simulink model "sampleModel20"  (R2021a)
settings: Solver=VariableStepAuto  StartTime=0.0  StopTime=10.0  RelTol=1e-3
undefined symbols (not defined in the file): DiscIntNeverNeededParam, magnitude, Newton, Raphson
libraries: simulink x274, pid_lib x17
(part 16 of 16)

== system sampleModel20/cfblk97/cfblk3/cfblk10/cfblk7 ==
  cfblk1 : Inport
  cfblk5 : Inport  Port=2
  cfblk6 : Inport  Port=3
  cfblk7 : Inport  Port=4
  cfblk8 : Inport  Port=5
  cfblk9 : Inport  Port=6
  cfblk10 : Inport  Port=7
  cfblk3 : Polyval  Coefs=[ +2.081618890e-019, -1.441693666e-014, +4.719686976e-010, -8.536869453e-006, +1.621573104e-001, -8.087801117e+001 ]
  cfblk4 : Signum
  cfblk2 : Outport
  cfblk11 : Outport  Port=2
  wires:
  cfblk8/1 -> cfblk3/1
  cfblk3/1 -> cfblk2/1
  cfblk4/1 -> cfblk11/1
  cfblk9/1 -> cfblk4/1

== system sampleModel20/cfblk97/cfblk3/cfblk5/cfblk10 ==
  cfblk1 : Inport
  cfblk8 : Inport  Port=2
  cfblk9 : Inport  Port=3
  cfblk10 : Inport  Port=4
  cfblk11 : Inport  Port=5
  cfblk12 : Inport  Port=6
  cfblk13 : Inport  Port=7
  cfblk3 : simulink/Discrete/Transfer Fcn Real Zero  ZeroZ=0.75  ICPrevInput=0.0  DoSatur=off
      settings: SourceProductBaseCode=SL
  cfblk4 : Gain  Gain=[233703993.927434]
  cfblk5 : Reshape
  cfblk6 : Signum
  cfblk7 : Bias  Bias=[437592239.040751]
  cfblk2 : Outport
  cfblk14 : Outport  Port=2
  cfblk15 : Outport  Port=3
  wires:
  cfblk7/1 -> cfblk5/1
  cfblk3/1 -> cfblk7/1
  cfblk1/1 -> cfblk15/1
  cfblk11/1 -> cfblk6/1
  cfblk8/1 -> cfblk4/1
  cfblk12/1 -> cfblk2/1
  cfblk4/1 -> cfblk14/1
  cfblk6/1 -> cfblk3/1

== system sampleModel20/cfblk97/cfblk3/cfblk5/cfblk11 ==
  cfblk1 : Inport
  cfblk6 : Inport  Port=2
  cfblk7 : Inport  Port=3
  cfblk8 : Inport  Port=4
  cfblk3 : simulink/Math Operations/Slider Gain  gain=1  low=0  high=2
  cfblk4 : Gain  Gain=[977320250.884013]
  cfblk5 : Gain  Gain=[-143070157.092891]
  cfblk2 : Outport
  cfblk9 : Outport  Port=2
  wires:
  cfblk8/1 -> cfblk9/1
  cfblk6/1 -> cfblk5/1
  cfblk5/1 -> cfblk4/1
  cfblk7/1 -> cfblk2/1
  cfblk1/1 -> cfblk3/1

== system sampleModel20/cfblk97/cfblk3/cfblk5/cfblk12 ==
  cfblk1 : Inport
  cfblk8 : Inport  Port=2
  cfblk9 : Inport  Port=3
  cfblk10 : Inport  Port=4
  cfblk11 : Inport  Port=5
  cfblk12 : Inport  Port=6
  cfblk13 : Inport  Port=7
  cfblk14 : Inport  Port=8
  cfblk3 : Polyval  Coefs=[ +2.081618890e-019, -1.441693666e-014, +4.719686976e-010, -8.536869453e-006, +1.621573104e-001, -8.087801117e+001 ]
  cfblk4 : Signum
  cfblk5 : Sqrt  Operator=rSqrt  AlgorithmType=Newton-Raphson  SaturateOnIntegerOverflow=on
  cfblk6 : PermuteDimensions
  cfblk7 : Reshape
  cfblk2 : Outport
  cfblk15 : Outport  Port=2
  cfblk16 : Outport  Port=3
  cfblk17 : Outport  Port=4
  wires:
  cfblk13/1 -> cfblk6/1
  cfblk10/1 -> cfblk7/1
  cfblk11/1 -> cfblk16/1
  cfblk6/1 -> cfblk15/1
  cfblk3/1 -> cfblk17/1
  cfblk8/1 -> cfblk3/1
  cfblk5/1 -> cfblk4/1
  cfblk1/1 -> cfblk2/1
  cfblk9/1 -> cfblk5/1

== system sampleModel20/cfblk97/cfblk3/cfblk5/cfblk7 ==
  cfblk1 : Inport
  cfblk6 : Inport  Port=2
  cfblk7 : Inport  Port=3
  cfblk8 : Inport  Port=4
  cfblk9 : Inport  Port=5
  cfblk10 : Inport  Port=6
  cfblk11 : Inport  Port=7
  cfblk12 : Inport  Port=8
  cfblk13 : Inport  Port=9
  cfblk14 : Inport  Port=10
  cfblk3 : Sqrt  SaturateOnIntegerOverflow=on
  cfblk4 : Sqrt  SaturateOnIntegerOverflow=on
  cfblk5 : Gain  Gain=[-337074961.948638]
  cfblk2 : Outport
  wires:
  cfblk4/1 -> cfblk5/1
  cfblk11/1 -> cfblk4/1
  cfblk14/1 -> cfblk3/1
  cfblk1/1 -> cfblk2/1

== system sampleModel20/cfblk97/cfblk3/cfblk5/cfblk8 ==
  cfblk1 : Inport
  cfblk8 : Inport  Port=2
  cfblk9 : Inport  Port=3
  cfblk10 : Inport  Port=4
  cfblk11 : Inport  Port=5
  cfblk12 : Inport  Port=6
  cfblk3 : Product
  cfblk4 : Squeeze
  cfblk5 : Trigonometry
  cfblk6 : Rounding
  cfblk7 : Product
  cfblk2 : Outport
  cfblk13 : Outport  Port=2
  cfblk14 : Outport  Port=3
  cfblk15 : Outport  Port=4
  wires:
  cfblk1/1 -> cfblk4/1
  cfblk7/1 -> cfblk14/1
  cfblk8/1 -> cfblk7/1
  cfblk5/1 -> cfblk7/2
  cfblk4/1 -> cfblk3/1
  cfblk10/1 -> cfblk5/1
  cfblk6/1 -> cfblk3/2
  cfblk12/1 -> cfblk6/1
  cfblk11/1 -> cfblk15/1
  cfblk3/1 -> cfblk2/1
  cfblk9/1 -> cfblk13/1

== system sampleModel20/cfblk97/cfblk3/cfblk5/cfblk9 ==
  cfblk1 : Inport
  cfblk8 : Inport  Port=2
  cfblk9 : Inport  Port=3
  cfblk10 : Inport  Port=4
  cfblk11 : Inport  Port=5
  cfblk12 : Inport  Port=6
  cfblk13 : Inport  Port=7
  cfblk3 : PermuteDimensions
  cfblk4 : ComplexToMagnitudeAngle
  cfblk5 : Sqrt  SaturateOnIntegerOverflow=on
  cfblk6 : Sum
  cfblk7 : simulink/Math Operations/MinMax Running Resettable  Function=min  vinit=0.0
  cfblk2 : Outport
  cfblk14 : Outport  Port=2
  wires:
  cfblk9/1 -> cfblk3/1
  cfblk11/1 -> cfblk6/1
  cfblk10/1 -> cfblk6/2
  cfblk1/1 -> cfblk4/1
  cfblk13/1 -> cfblk7/1
  cfblk12/1 -> cfblk14/1
  cfblk3/1 -> cfblk2/1
  cfblk8/1 -> cfblk7/2
  cfblk6/1 -> cfblk5/1

== system sampleModel20/cfblk97/cfblk3/cfblk6/cfblk10 ==
  cfblk1 : Inport
  cfblk4 : Inport  Port=2
  cfblk5 : Inport  Port=3
  cfblk6 : Inport  Port=4
  cfblk7 : Inport  Port=5
  cfblk8 : Inport  Port=6
  cfblk9 : Inport  Port=7
  cfblk3 : Sin  TimeSource=Use external signal  SampleTime=0
  cfblk2 : Outport
  wires:
  cfblk1/1 -> cfblk3/1
  cfblk9/1 -> cfblk2/1

== system sampleModel20/cfblk97/cfblk3/cfblk6/cfblk11 ==
  cfblk1 : Inport
  cfblk8 : Inport  Port=2
  cfblk9 : Inport  Port=3
  cfblk10 : Inport  Port=4
  cfblk11 : Inport  Port=5
  cfblk3 : MinMax  Function=max  Inputs=2
  cfblk4 : ComplexToRealImag
  cfblk5 : Abs
  cfblk6 : ComplexToMagnitudeAngle
  cfblk7 : Sum  Inputs=+
  cfblk2 : Outport
  cfblk12 : Outport  Port=2
  cfblk13 : Outport  Port=3
  wires:
  cfblk10/1 -> cfblk2/1
  cfblk3/1 -> cfblk5/1
  cfblk6/1 -> cfblk4/1
  cfblk6/2 -> cfblk7/1
  cfblk11/1 -> cfblk12/1
  cfblk1/1 -> cfblk3/1
  cfblk7/1 -> cfblk13/1
  cfblk9/1 -> cfblk6/1
  cfblk8/1 -> cfblk3/2

== system sampleModel20/cfblk97/cfblk3/cfblk6/cfblk12 ==
  cfblk1 : Inport
  cfblk6 : Inport  Port=2
  cfblk7 : Inport  Port=3
  cfblk8 : Inport  Port=4
  cfblk9 : Inport  Port=5
  cfblk3 : Sqrt  Operator=rSqrt  AlgorithmType=Newton-Raphson  SaturateOnIntegerOverflow=on
  cfblk4 : MinMax
  cfblk5 : Signum
  cfblk2 : Outport
  wires:
  cfblk5/1 -> cfblk2/1
  cfblk9/1 -> cfblk4/1
  cfblk8/1 -> cfblk3/1
  cfblk3/1 -> cfblk5/1

== system sampleModel20/cfblk97/cfblk3/cfblk6/cfblk8 ==
  cfblk1 : Inport
  cfblk5 : Inport  Port=2
  cfblk6 : Inport  Port=3
  cfblk7 : Inport  Port=4
  cfblk3 : PermuteDimensions
  cfblk4 : DotProduct  InputSameDT=on  OutDataTypeStr=Inherit: Inherit via internal rule
  cfblk2 : Outport
  wires:
  cfblk4/1 -> cfblk3/1
  cfblk6/1 -> cfblk4/1
  cfblk1/1 -> cfblk4/2
  cfblk7/1 -> cfblk2/1

== system sampleModel20/cfblk97/cfblk3/cfblk6/cfblk9 ==
  cfblk1 : Inport
  cfblk10 : Inport  Port=2
  cfblk11 : Inport  Port=3
  cfblk12 : Inport  Port=4
  cfblk15 : Delay  SampleTime=1
  cfblk16 : Delay  SampleTime=1
  cfblk3 : Bias  Bias=[-118316642.771134]
  cfblk4 : ComplexToMagnitudeAngle
  cfblk5 : ComplexToMagnitudeAngle
  cfblk6 : Assignment  DiagnosticForDimensions=Warning  IndexOptions=Index vector (dialog)  Indices=1  OutputSizes=1
  cfblk7 : DotProduct  InputSameDT=on  OutDataTypeStr=Inherit: Inherit via internal rule
  cfblk8 : Assignment  DiagnosticForDimensions=Warning  IndexOptions=Index vector (dialog)  Indices=1  OutputSizes=1
  cfblk9 : Sqrt  Operator=rSqrt  AlgorithmType=Newton-Raphson  SaturateOnIntegerOverflow=on
  cfblk2 : Outport
  cfblk13 : Outport  Port=2
  cfblk14 : Outport  Port=3
  wires:
  cfblk11/1 -> cfblk7/1
  cfblk9/1 -> cfblk2/1
  cfblk4/1 -> cfblk13/1
  cfblk1/1 -> cfblk9/1
  cfblk10/1 -> cfblk14/1
  cfblk6/1 -> cfblk5/1
  cfblk12/1 -> cfblk4/1
  cfblk3/1 -> cfblk7/2
  cfblk7/1 -> cfblk6/1
  cfblk5/2 -> cfblk8/2, cfblk16/1
  cfblk4/2 -> cfblk8/1
  cfblk5/1 -> cfblk15/1
  cfblk15/1 -> cfblk3/1
  cfblk16/1 -> cfblk6/2

== system sampleModel20/cfblk97/cfblk3/cfblk7/cfblk5 ==
  cfblk1 : Inport
  cfblk8 : Inport  Port=2
  cfblk9 : Inport  Port=3
  cfblk10 : Inport  Port=4
  cfblk11 : Inport  Port=5
  cfblk3 : Product
  cfblk4 : Sum  Inputs=|++
  cfblk5 : Trigonometry
  cfblk6 : Squeeze
  cfblk7 : Sin  TimeSource=Use external signal  SampleTime=0
  cfblk2 : Outport
  cfblk12 : Outport  Port=2
  wires:
  cfblk10/1 -> cfblk7/1
  cfblk5/1 -> cfblk6/1
  cfblk9/1 -> cfblk5/1
  cfblk11/1 -> cfblk3/1
  cfblk7/1 -> cfblk12/1
  cfblk1/1 -> cfblk3/2
  cfblk8/1 -> cfblk4/1
  cfblk6/1 -> cfblk4/2
  cfblk3/1 -> cfblk2/1

== system sampleModel20/cfblk97/cfblk3/cfblk7/cfblk6 ==
  cfblk1 : Inport
  cfblk7 : Inport  Port=2
  cfblk8 : Inport  Port=3
  cfblk9 : Inport  Port=4
  cfblk10 : Inport  Port=5
  cfblk11 : Inport  Port=6
  cfblk12 : Inport  Port=7
  cfblk13 : Delay  SampleTime=1
  cfblk3 : Product  Inputs=**
  cfblk4 : Product  Inputs=**
  cfblk5 : Polyval  Coefs=[ +2.081618890e-019, -1.441693666e-014, +4.719686976e-010, -8.536869453e-006, +1.621573104e-001, -8.087801117e+001 ]
  cfblk6 : simulink/Math Operations/MinMax Running Resettable  Function=min  vinit=0.0
  cfblk2 : Outport
  wires:
  cfblk4/1 -> cfblk5/1
  cfblk1/1 -> cfblk6/1
  cfblk10/1 -> cfblk2/1
  cfblk3/1 -> cfblk4/2
  cfblk8/1 -> cfblk3/1
  cfblk11/1 -> cfblk6/2
  cfblk6/1 -> cfblk3/2
  cfblk5/1 -> cfblk13/1
  cfblk13/1 -> cfblk4/1

== system sampleModel20/cfblk97/cfblk3/cfblk8/cfblk5 ==
  cfblk1 : Inport
  cfblk9 : Inport  Port=2
  cfblk10 : Inport  Port=3
  cfblk11 : Inport  Port=4
  cfblk12 : Inport  Port=5
  cfblk13 : Inport  Port=6
  cfblk14 : Inport  Port=7
  cfblk15 : Inport  Port=8
  cfblk3 : Bias  Bias=[-928237704.181962]
  cfblk4 : Rounding
  cfblk5 : Product  Inputs=**
  cfblk6 : Sum
  cfblk7 : Trigonometry
  cfblk8 : Sin  TimeSource=Use external signal  SampleTime=0
  cfblk2 : Outport
  cfblk16 : Outport  Port=2
  wires:
  cfblk11/1 -> cfblk16/1
  cfblk3/1 -> cfblk5/1
  cfblk9/1 -> cfblk4/1
  cfblk4/1 -> cfblk6/1
  cfblk6/1 -> cfblk7/1
  cfblk14/1 -> cfblk6/2
  cfblk10/1 -> cfblk5/2
  cfblk8/1 -> cfblk2/1
  cfblk12/1 -> cfblk3/1
  cfblk7/1 -> cfblk8/1

== system sampleModel20/cfblk97/cfblk3/cfblk8/cfblk6 ==
  cfblk1 : Inport
  cfblk9 : Inport  Port=2
  cfblk10 : Inport  Port=3
  cfblk11 : Inport  Port=4
  cfblk12 : Inport  Port=5
  cfblk13 : Inport  Port=6
  cfblk14 : Inport  Port=7
  cfblk3 : Math  Operator=transpose  SaturateOnIntegerOverflow=on
  cfblk4 : Math  Operator=transpose  SaturateOnIntegerOverflow=on
  cfblk5 : Math  Operator=mod  SaturateOnIntegerOverflow=on
  cfblk6 : Math  Operator=pow  SaturateOnIntegerOverflow=on
  cfblk7 : Abs
  cfblk8 : UnaryMinus
  cfblk2 : Outport
  wires:
  cfblk3/1 -> cfblk2/1
  cfblk11/1 -> cfblk5/1
  cfblk14/1 -> cfblk8/1
  cfblk9/1 -> cfblk3/1
  cfblk1/1 -> cfblk5/2
  cfblk6/1 -> cfblk4/1
  cfblk8/1 -> cfblk7/1
  cfblk7/1 -> cfblk6/1
  cfblk13/1 -> cfblk6/2

== system sampleModel20/cfblk97/cfblk3/cfblk9/cfblk10 ==
  cfblk1 : Inport
  cfblk10 : Inport  Port=2
  cfblk11 : Inport  Port=3
  cfblk12 : Inport  Port=4
  cfblk13 : Delay  SampleTime=1
  cfblk3 : Sqrt  Operator=rSqrt  AlgorithmType=Newton-Raphson  SaturateOnIntegerOverflow=on
  cfblk4 : Sin  TimeSource=Use external signal  SampleTime=0
  cfblk5 : UnaryMinus
  cfblk6 : Product
  cfblk7 : simulink/Math Operations/MinMax Running Resettable  Function=min  vinit=0.0
  cfblk8 : UnaryMinus
  cfblk9 : Product
  cfblk2 : Outport
  wires:
  cfblk11/1 -> cfblk6/1
  cfblk6/1 -> cfblk7/1
  cfblk8/1 -> cfblk9/1
  cfblk1/1 -> cfblk7/2
  cfblk12/1 -> cfblk5/1
  cfblk5/1 -> cfblk6/2
  cfblk9/1 -> cfblk4/1
  cfblk7/1 -> cfblk2/1
  cfblk10/1 -> cfblk8/1
  cfblk3/1 -> cfblk9/2
  cfblk4/1 -> cfblk13/1
  cfblk13/1 -> cfblk3/1

== system sampleModel20/cfblk97/cfblk3/cfblk9/cfblk11 ==
  cfblk1 : Inport
  cfblk8 : Inport  Port=2
  cfblk3 : Trigonometry
  cfblk4 : ComplexToMagnitudeAngle
  cfblk5 : ComplexToRealImag
  cfblk6 : Rounding
  cfblk7 : Sum
  cfblk2 : Outport
  wires:
  cfblk1/1 -> cfblk3/1
  cfblk3/1 -> cfblk4/1
  cfblk4/1 -> cfblk5/1
  cfblk5/1 -> cfblk6/1
  cfblk4/2 -> cfblk7/1
  cfblk5/2 -> cfblk2/1
  cfblk8/1 -> cfblk7/2

== system sampleModel20/cfblk97/cfblk3/cfblk9/cfblk12 ==
  cfblk1 : Inport
  cfblk7 : Inport  Port=2
  cfblk8 : Inport  Port=3
  cfblk9 : Inport  Port=4
  cfblk10 : Inport  Port=5
  cfblk11 : Inport  Port=6
  cfblk12 : Inport  Port=7
  cfblk3 : Bias  Bias=[-457409305.368843]
  cfblk4 : Product  Inputs=*
  cfblk5 : Product
  cfblk6 : Sqrt  Operator=rSqrt  AlgorithmType=Newton-Raphson  SaturateOnIntegerOverflow=on
  cfblk2 : Outport
  cfblk13 : Outport  Port=2
  wires:
  cfblk10/1 -> cfblk13/1
  cfblk12/1 -> cfblk4/1
  cfblk4/1 -> cfblk3/1
  cfblk1/1 -> cfblk6/1
  cfblk11/1 -> cfblk5/1
  cfblk7/1 -> cfblk2/1
  cfblk8/1 -> cfblk5/2

== system sampleModel20/cfblk97/cfblk3/cfblk9/cfblk13 ==
  cfblk1 : Inport
  cfblk8 : Inport  Port=2
  cfblk11 : Delay  SampleTime=1
  cfblk12 : Delay  SampleTime=1
  cfblk3 : UnaryMinus
  cfblk4 : Sum  Inputs=+-
  cfblk5 : PermuteDimensions
  cfblk6 : ComplexToRealImag
  cfblk7 : Sum  Inputs=|++
  cfblk2 : Outport
  cfblk9 : Outport  Port=2
  cfblk10 : Outport  Port=3
  wires:
  cfblk5/1 -> cfblk2/1, cfblk12/1
  cfblk3/1 -> cfblk7/1
  cfblk8/1 -> cfblk6/1
  cfblk6/1 -> cfblk4/1
  cfblk7/1 -> cfblk4/2
  cfblk4/1 -> cfblk5/1, cfblk11/1
  cfblk1/1 -> cfblk10/1
  cfblk6/2 -> cfblk9/1
  cfblk11/1 -> cfblk7/2
  cfblk12/1 -> cfblk3/1

== system sampleModel20/cfblk97/cfblk4/cfblk4/cfblk10 ==
  cfblk1 : Inport
  cfblk7 : Inport  Port=2
  cfblk8 : Inport  Port=3
  cfblk9 : Inport  Port=4
  cfblk10 : Inport  Port=5
  cfblk11 : Inport  Port=6
  cfblk12 : Inport  Port=7
  cfblk3 : Bias  Bias=[-722433701.739389]
  cfblk4 : DotProduct  InputSameDT=on  OutDataTypeStr=Inherit: Inherit via internal rule
  cfblk5 : Product
  cfblk6 : Product  Inputs=**
  cfblk2 : Outport
  wires:
  cfblk9/1 -> cfblk6/1
  cfblk5/1 -> cfblk3/1
  cfblk11/1 -> cfblk4/1
  cfblk3/1 -> cfblk6/2
  cfblk4/1 -> cfblk5/1
  cfblk1/1 -> cfblk2/1
  cfblk12/1 -> cfblk5/2
  cfblk8/1 -> cfblk4/2

== system sampleModel20/cfblk97/cfblk4/cfblk4/cfblk11 ==
  cfblk1 : Inport
  cfblk6 : Inport  Port=2
  cfblk7 : Inport  Port=3
  cfblk8 : Inport  Port=4
  cfblk9 : Inport  Port=5
  cfblk10 : Inport  Port=6
  cfblk11 : Inport  Port=7
  cfblk12 : Inport  Port=8
  cfblk13 : Inport  Port=9
  cfblk14 : Inport  Port=10
  cfblk3 : Sum  Inputs=+-
  cfblk4 : simulink/Math Operations/Slider Gain  gain=1  low=0  high=2
  cfblk5 : Product
  cfblk2 : Outport
  wires:
  cfblk14/1 -> cfblk4/1
  cfblk4/1 -> cfblk5/1
  cfblk9/1 -> cfblk2/1
  cfblk8/1 -> cfblk3/1
  cfblk3/1 -> cfblk5/2
  cfblk12/1 -> cfblk3/2

== system sampleModel20/cfblk97/cfblk4/cfblk4/cfblk12 ==
  cfblk1 : Inport
  cfblk5 : Inport  Port=2
  cfblk6 : Inport  Port=3
  cfblk7 : Inport  Port=4
  cfblk8 : Inport  Port=5
  cfblk3 : Signum
  cfblk4 : Abs
  cfblk2 : Outport
  cfblk9 : Outport  Port=2
  wires:
  cfblk5/1 -> cfblk3/1
  cfblk6/1 -> cfblk4/1
  cfblk4/1 -> cfblk2/1
  cfblk1/1 -> cfblk9/1

== system sampleModel20/cfblk97/cfblk4/cfblk4/cfblk13 ==
  cfblk1 : Inport
  cfblk12 : Inport  Port=2
  cfblk13 : Inport  Port=3
  cfblk14 : Inport  Port=4
  cfblk15 : Inport  Port=5
  cfblk16 : Inport  Port=6
  cfblk10 : PermuteDimensions
  cfblk11 : Assignment  DiagnosticForDimensions=Warning  IndexOptions=Index vector (dialog)  Indices=1  OutputSizes=1
  cfblk18 : Delay  SampleTime=1
  cfblk3 : simulink/Discrete/Tapped Delay  vinit=0.0  samptime=-1  NumDelays=1  DelayOrder=Oldest  includeCurrent=off
  cfblk4 : ComplexToMagnitudeAngle
  cfblk5 : UnaryMinus
  cfblk6 : Gain  Gain=[836880504.048607]
  cfblk7 : PermuteDimensions
  cfblk8 : Sum  Inputs=+-
  cfblk9 : Assignment  DiagnosticForDimensions=Warning  IndexOptions=Index vector (dialog)  Indices=1  OutputSizes=1
  cfblk2 : Outport
  cfblk17 : Outport  Port=2
  wires:
  cfblk14/1 -> cfblk4/1
  cfblk5/1 -> cfblk6/1
  cfblk16/1 -> cfblk7/1
  cfblk8/1 -> cfblk17/1
  cfblk15/1 -> cfblk10/1
  cfblk12/1 -> cfblk8/1
  cfblk7/1 -> cfblk2/1
  cfblk13/1 -> cfblk8/2
  cfblk11/1 -> cfblk5/1
  cfblk10/1 -> cfblk11/1
  cfblk3/1 -> cfblk11/2
  cfblk6/1 -> cfblk9/1
  cfblk4/1 -> cfblk9/2
  cfblk9/1 -> cfblk18/1
  cfblk18/1 -> cfblk3/1

== system sampleModel20/cfblk97/cfblk4/cfblk4/cfblk8 ==
  cfblk1 : Inport
  cfblk6 : Inport  Port=2
  cfblk3 : pid_lib/PID Controller  Controller=PID  Form=Parallel  TimeDomain=Discrete-time  UseExternalTs=off  SampleTime=1  IntegratorMethod=Forward Euler  FilterMethod=Forward Euler  ControllerParametersSource=internal  P=1  I=1  D=0  UseFilter=on  N=100  TunerSelectOption=Transfer Function Based (PID Tuner App)  InitialConditionSource=internal  InitialConditionForIntegrator=0  InitialConditionForFilter=0  DifferentiatorICPrevScaledInput=0  ExternalReset=none  TrackingMode=off  Kt=1  LimitOutput=off  SatLimitsSource=internal  UpperSaturationLimit=inf  LowerSaturationLimit=-inf  LinearizeAsGain=off  AntiWindupMode=none  Kb=1  POutMin=[]  POutMax=[]  IOutMin=[]  IOutMax=[]  DOutMin=[]  DOutMax=[]  NOutMin=[]  NOutMax=[]  SumOutMin=[]  SumOutMax=[]  SaturationOutMin=[]  SaturationOutMax=[]  PParamMin=[]  PParamMax=[]  IParamMin=[]  IParamMax=[]  DParamMin=[]  DParamMax=[]  NParamMin=[]  NParamMax=[]  KbParamMin=[]  KbParamMax=[]  KtParamMin=[]  KtParamMax=[]  KbOutMin=[]  KbOutMax=[]  KtOutMin=[]  KtOutMax=[]  IntegratorOutMin=[]  IntegratorOutMax=[]  FilterOutMin=[]  FilterOutMax=[]  SumI1OutMin=[]  SumI1OutMax=[]  SumI2OutMin=[]  SumI2OutMax=[]  SumI3OutMin=[]  SumI3OutMax=[]  SumI4OutMin=[]  SumI4OutMax=[]  SumDOutMin=[]  SumDOutMax=[]  DifferentiatorOutMin=[]  DifferentiatorOutMax=[]  FilterDiffOutCoefMin=[]  FilterDiffOutCoefMax=[]  ReciprocalOutMin=[]  ReciprocalOutMax=[]  SumDenOutMin=[]  SumDenOutMax=[]  SumNumOutMin=[]  SumNumOutMax=[]  DivideOutMin=[]  DivideOutMax=[]  UdiffTsProdOutMin=[]  UdiffTsProdOutMax=[]  NTsProdOutMin=[]  NTsProdOutMax=[]  UintegralTsProdOutMin=[]  UintegralTsProdOutMax=[]  UngainTsProdOutMin=[]  UngainTsProdOutMax=[]  IntegratorContinuousStateAttributes=''  IntegratorStateMustResolveToSignalObject=off  IntegratorRTWStateStorageClass=Auto  FilterContinuousStateAttributes=''  FilterStateMustResolveToSignalObject=off  FilterRTWStateStorageClass=Auto  ParallelPVariant=InternalParameters  IdealPVariant=Disabled  IVariant=InternalParameters  DVariant=InternalParameters  IntegratorVariant=Discrete  SatVariant=Disabled  AWVariant=Passthrough  PCopyVariant=Disabled  TRVariant=Disabled  FdbkBlocksVariant=Forward  IdealPFdbkVariant=Disabled  SatFdbkVariant=Disabled  DerivativeFilterVariant=ForwardEulerFilter  NVariant=InternalParameters  NCopyVariant=Disabled  FilterICVariant=InternalICsFilter  IntegratorICVariant=InternalICs  ExternalResetVariant=Disabled  TRSumVariant=Passthrough  SumFdbkVariant=Disabled  SumVariant=Sum_PID  TsampFilterVariant=InternalTs  TsampNgainVariant=Passthrough  TsampIntegralVariant=Passthrough  ExternalSaturationOutDataTypeStr=Inherit: Same as second input
  cfblk4 : simulink/Discrete/Transfer Fcn First Order  PoleZ=0.95  ICPrevOutput=0.0  DoSatur=off
  cfblk5 : Math  Operator=log10  SaturateOnIntegerOverflow=on
  cfblk2 : Outport
  cfblk7 : Outport  Port=2
  wires:
  cfblk4/1 -> cfblk5/1
  cfblk6/1 -> cfblk7/1
  cfblk1/1 -> cfblk4/1
  cfblk5/1 -> cfblk3/1
  cfblk3/1 -> cfblk2/1

== system sampleModel20/cfblk97/cfblk4/cfblk4/cfblk9 ==
  cfblk1 : Inport
  cfblk5 : Inport  Port=2
  cfblk6 : Inport  Port=3
  cfblk7 : Inport  Port=4
  cfblk8 : Inport  Port=5
  cfblk9 : Inport  Port=6
  cfblk10 : Inport  Port=7
  cfblk3 : simulink/Math Operations/Slider Gain  gain=1  low=0  high=2
  cfblk4 : DotProduct  InputSameDT=on  OutDataTypeStr=Inherit: Inherit via internal rule
  cfblk2 : Outport
  cfblk11 : Outport  Port=2
  cfblk12 : Outport  Port=3
  cfblk13 : Outport  Port=4
  wires:
  cfblk8/1 -> cfblk11/1
  cfblk5/1 -> cfblk2/1
  cfblk6/1 -> cfblk4/1
  cfblk9/1 -> cfblk3/1
  cfblk10/1 -> cfblk4/2
  cfblk4/1 -> cfblk13/1
  cfblk7/1 -> cfblk12/1

== system sampleModel20/cfblk97/cfblk4/cfblk6/cfblk7 ==
  cfblk1 : Inport
  cfblk7 : Inport  Port=2
  cfblk8 : Inport  Port=3
  cfblk9 : Inport  Port=4
  cfblk10 : Inport  Port=5
  cfblk11 : Inport  Port=6
  cfblk12 : Inport  Port=7
  cfblk3 : Abs
  cfblk4 : Sqrt  SaturateOnIntegerOverflow=on
  cfblk5 : ComplexToRealImag
  cfblk6 : Sqrt  Operator=rSqrt  AlgorithmType=Newton-Raphson  SaturateOnIntegerOverflow=on
  cfblk2 : Outport
  cfblk13 : Outport  Port=2
  cfblk14 : Outport  Port=3
  cfblk15 : Outport  Port=4
  cfblk16 : Outport  Port=5
  wires:
  cfblk4/1 -> cfblk6/1
  cfblk6/1 -> cfblk16/1
  cfblk9/1 -> cfblk3/1
  cfblk5/1 -> cfblk13/1
  cfblk3/1 -> cfblk5/1
  cfblk5/2 -> cfblk15/1
  cfblk1/1 -> cfblk4/1
  cfblk10/1 -> cfblk14/1
  cfblk7/1 -> cfblk2/1

== system sampleModel20/cfblk97/cfblk4/cfblk6/cfblk8 ==
  cfblk1 : Inport
  cfblk8 : Inport  Port=2
  cfblk9 : Inport  Port=3
  cfblk10 : Inport  Port=4
  cfblk11 : Inport  Port=5
  cfblk12 : Inport  Port=6
  cfblk13 : Inport  Port=7
  cfblk14 : Inport  Port=8
  cfblk3 : DotProduct  InputSameDT=on  OutDataTypeStr=Inherit: Inherit via internal rule
  cfblk4 : Squeeze
  cfblk5 : Abs
  cfblk6 : Product  Inputs=**
  cfblk7 : Sqrt  Operator=rSqrt  AlgorithmType=Newton-Raphson  SaturateOnIntegerOverflow=on
  cfblk2 : Outport
  cfblk15 : Outport  Port=2
  wires:
  cfblk3/1 -> cfblk7/1
  cfblk13/1 -> cfblk2/1
  cfblk5/1 -> cfblk15/1
  cfblk9/1 -> cfblk3/1
  cfblk12/1 -> cfblk4/1
  cfblk8/1 -> cfblk6/1
  cfblk14/1 -> cfblk6/2
  cfblk4/1 -> cfblk3/2
  cfblk10/1 -> cfblk5/1
